simulink subsystem "SenalizadorAj"  (R2023b)
settings: Solver=VariableStepAuto  StartTime=0.0  StopTime=10.0  RelTol=1e-3
libraries: simulink x8
settings Model: Creator=USUARIO  LastModifiedBy=USUARIO

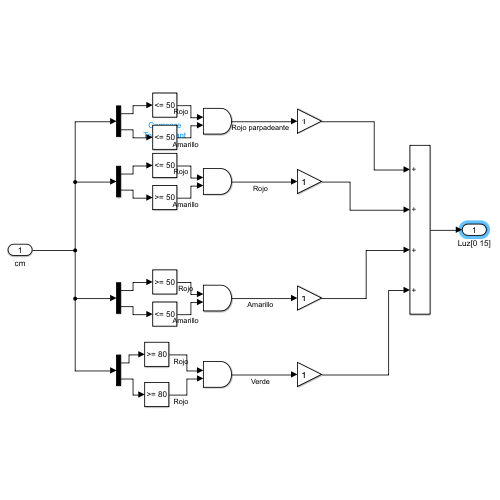
[thumbnail: Simulink's stored preview of the top-level diagram]
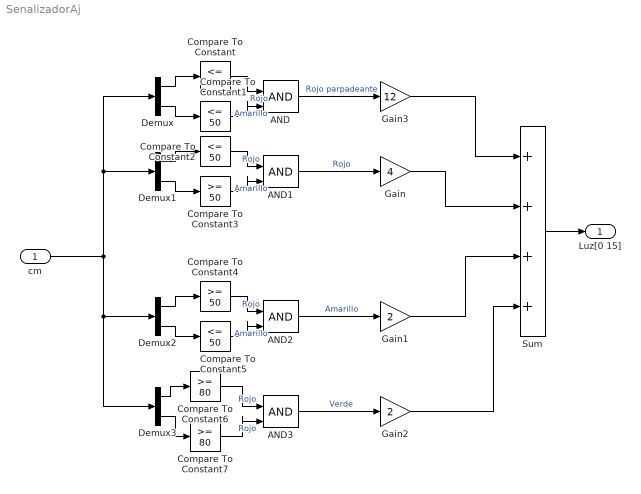
== system SenalizadorAj ==
  cm : Inport
  AND{,1..3} (4 alike) : Logic  IconShape=distinctive  AllPortsSameDT=off  OutDataTypeStr=boolean
  Compare To Constant{,1..2,5} (4 alike) : simulink/Logic and Bit Operations/Compare To Constant  relop=<=  const=50  OutDataTypeStr=boolean
  Compare To Constant3 : simulink/Logic and Bit Operations/Compare To Constant  relop=>=  const=50  OutDataTypeStr=boolean
  Compare To Constant4 : simulink/Logic and Bit Operations/Compare To Constant  relop=>=  const=50  OutDataTypeStr=boolean
  Compare To Constant6 : simulink/Logic and Bit Operations/Compare To Constant  relop=>=  const=80  OutDataTypeStr=boolean
  Compare To Constant7 : simulink/Logic and Bit Operations/Compare To Constant  relop=>=  const=80  OutDataTypeStr=boolean
  Demux{,1..3} (4 alike) : Demux  Outputs=2
  Gain : Gain  Gain=4  OutDataTypeStr=int16
  Gain1 : Gain  Gain=2  OutDataTypeStr=int16
  Gain2 : Gain  Gain=2  OutDataTypeStr=int16
  Gain3 : Gain  Gain=12  OutDataTypeStr=int16
  Sum : Sum  Inputs=++++
  Luz[0 15] : Outport
  wires:
  cm/1 -> Demux1/1, Demux/1, Demux3/1, Demux2/1
  Demux/2 -> Compare To Constant1/1
  Demux/1 -> Compare To Constant/1
  Compare To Constant/1 -> AND/1  "Rojo"
  Compare To Constant1/1 -> AND/2  "Amarillo"
  Compare To Constant2/1 -> AND1/1  "Rojo"
  Demux1/1 -> Compare To Constant2/1
  Compare To Constant3/1 -> AND1/2  "Amarillo"
  Demux1/2 -> Compare To Constant3/1
  Compare To Constant4/1 -> AND2/1  "Rojo"
  Demux2/1 -> Compare To Constant4/1
  Compare To Constant5/1 -> AND2/2  "Amarillo"
  Demux2/2 -> Compare To Constant5/1
  Demux3/1 -> Compare To Constant6/1
  Demux3/2 -> Compare To Constant7/1
  Compare To Constant6/1 -> AND3/1  "Rojo"
  Compare To Constant7/1 -> AND3/2  "Rojo"
  AND/1 -> Gain3/1  "Rojo parpadeante"
  AND1/1 -> Gain/1  "Rojo"
  AND2/1 -> Gain1/1  "Amarillo"
  AND3/1 -> Gain2/1  "Verde"
  Gain3/1 -> Sum/1
  Gain/1 -> Sum/2
  Gain1/1 -> Sum/3
  Gain2/1 -> Sum/4
  Sum/1 -> Luz[0 15]/1
